simulink model "mobilebot_Model"  (R2018a)
settings: Solver=VariableStepAuto  StartTime=0.0  StopTime=10.0  RelTol=1e-3
libraries: simulink x2
settings Model: Creator=ewolbrec  LastModifiedBy=nalha
settings CodeAppCC: StateflowObjectComments=on

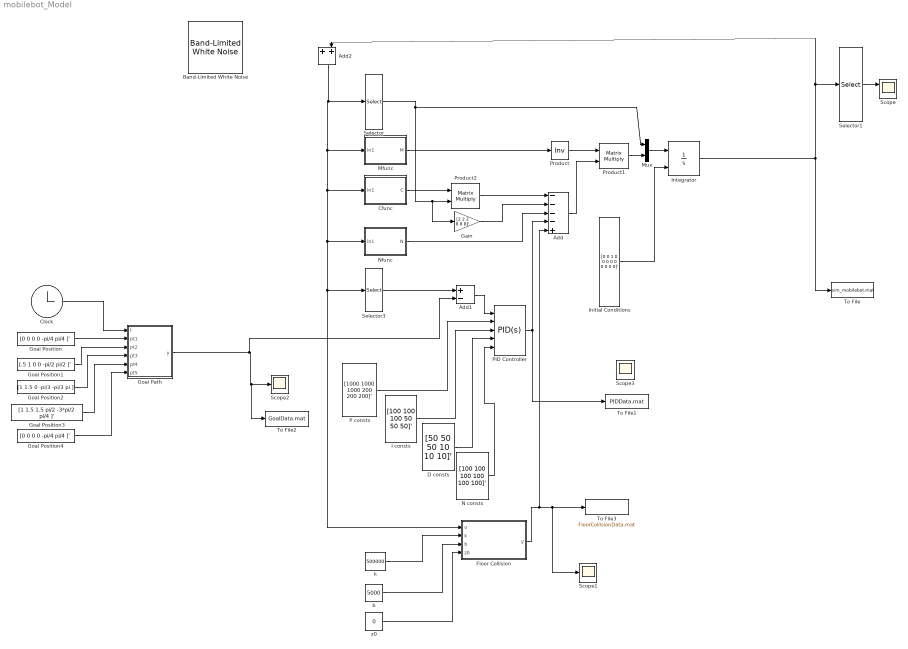
== system mobilebot_Model ==
  Add : Sum  Inputs=----+
  Add1 : Sum  Inputs=+-
  Add2 : Sum
  Band-Limited White Noise : simulink/Sources/Band-Limited White Noise  Cov=[0.00001 0.00001 0.0 0.00001 0.00001 0.00001 0.00001 0.00001 0.00001 0.00001 0.00001 0.00001]  Ts=1/30  seed=[23341 45275 30585 21083 69043 57234 42583 21474 10234 94373 48378 902740]
  Cfunc : MATLAB Function  TreatAsAtomicUnit=on
  Clock : Clock
  D consts : Constant  Value=[50 50 50 10 10 10]'  VectorParams1D=off
  Floor Collision : MATLAB Function  TreatAsAtomicUnit=on
  Gain : Gain  Gain=[2 2 2 8 8 8]'
  Goal Path : MATLAB Function  TreatAsAtomicUnit=on
  Goal Position : Constant  Value=[0 0 0 0 -pi/4 pi/4 ]'  VectorParams1D=off
  Goal Position1 : Constant  Value=[.5 1 0 0 -pi/2 pi/2 ]'  VectorParams1D=off
  Goal Position2 : Constant  Value=[1 1.5 0 -pi/3 -pi/3 pi ]'  VectorParams1D=off
  Goal Position3 : Constant  Value=[1 1.5 1.5 pi/2 -3*pi/2 pi/4 ]'  VectorParams1D=off
  Goal Position4 : Constant  Value=[0 0 0 0 -pi/4 pi/4 ]'  VectorParams1D=off
  I consts : Constant  Value=[100 100 100 50 50 50]'  VectorParams1D=off
  Initial Conditions : Constant  Value=[0 0 1 0 0 0 0 0 0 0 0 0]'  VectorParams1D=off
  Integrator : Integrator  InitialConditionSource=external
  Mfunc : MATLAB Function  TreatAsAtomicUnit=on
  Mux : Mux  Inputs=2
  N consts : Constant  Value=[100 100 100 100 100 100]'  VectorParams1D=off
  Nfunc : MATLAB Function  TreatAsAtomicUnit=on
  P consts : Constant  Value=[1000 1000 1000 200 200 200]'  VectorParams1D=off
  PID Controller : simulink/Continuous/PID Controller  Controller=PID  TimeDomain=Continuous-time  SampleTime=-1  IntegratorMethod=Forward Euler  FilterMethod=Forward Euler  Form=Parallel  UseFilter=on  ControllerParametersSource=external  P=200  I=25  D=70  N=150  InitialConditionSource=internal  InitialConditionForIntegrator=0  InitialConditionForFilter=0  ExternalReset=none  LimitOutput=off  UpperSaturationLimit=inf  LowerSaturationLimit=-inf  LinearizeAsGain=on  AntiWindupMode=none  Kb=1  TrackingMode=off  Kt=1  PParamMin=[]  PParamMax=[]  IParamMin=[]  IParamMax=[]  DParamMin=[]  DParamMax=[]  NParamMin=[]  NParamMax=[]  KbParamMin=[]  KbParamMax=[]  KtParamMin=[]  KtParamMax=[]  POutMin=[]  POutMax=[]  IOutMin=[]  IOutMax=[]  DOutMin=[]  DOutMax=[]  NOutMin=[]  NOutMax=[]  KbOutMin=[]  KbOutMax=[]  KtOutMin=[]  KtOutMax=[]  IntegratorOutMin=[]  IntegratorOutMax=[]  FilterOutMin=[]  FilterOutMax=[]  SumOutMin=[]  SumOutMax=[]  SumI1OutMin=[]  SumI1OutMax=[]  SumI2OutMin=[]  SumI2OutMax=[]  SumI3OutMin=[]  SumI3OutMax=[]  SumDOutMin=[]  SumDOutMax=[]  SaturationOutMin=[]  SaturationOutMax=[]  IntegratorContinuousStateAttributes=''  IntegratorStateMustResolveToSignalObject=off  IntegratorRTWStateStorageClass=Auto  FilterContinuousStateAttributes=''  FilterStateMustResolveToSignalObject=off  FilterRTWStateStorageClass=Auto  DifferentiatorICPrevScaledInput=0  DifferentiatorOutMin=[]  DifferentiatorOutMax=[]  FilterDiffOutCoefMin=[]  FilterDiffOutCoefMax=[]  SumDenOutMin=[]  SumDenOutMax=[]  SumNumOutMin=[]  SumNumOutMax=[]  ReciprocalOutMin=[]  ReciprocalOutMax=[]  DivideOutMin=[]  DivideOutMax=[]  TunerSelectOption=Transfer Function Based (PID Tuner App)
  Product : Product  Inputs=/  Multiplication=Matrix(*)
  Product1 : Product  Inputs=**  Multiplication=Matrix(*)
  Product2 : Product  Inputs=**  Multiplication=Matrix(*)
  Scope : Scope  NumInputPorts=2
  Scope1 : Scope
  Scope2 : Scope
  Scope3 : Scope
  Selector : Selector  InputPortWidth=12  IndexOptions=Index vector (dialog)  Indices=[7 8 9 10 11 12]  OutputSizes=1
  Selector1 : Selector  InputPortWidth=12  IndexOptions=Index vector (dialog)  Indices=[1 2 3 4 5 6]  OutputSizes=1
  Selector3 : Selector  InputPortWidth=12  IndexOptions=Index vector (dialog)  Indices=[1 2 3 4 5 6]  OutputSizes=1
  To File : ToFile  Filename=sim_mobilebot.mat  SampleTime=1/30
  To File1 : ToFile  Filename=PIDData.mat  SampleTime=1/30
  To File2 : ToFile  Filename=GoalData.mat  SampleTime=1/30
  To File3 : ToFile  Filename=FloorCollisionData.mat  SampleTime=1/30
  "b " : Constant  Value=5000
  "k " : Constant  Value=500000
  z0 : Constant  Value=0
  wires:
  Mfunc/1(M) -> Product/1
  Mux/1 -> Integrator/1
  Product1/1 -> Mux/2
  Selector/1 -> Gain/1, Product2/2, Mux/1
  Cfunc/1(C) -> Product2/1
  Product/1 -> Product1/1
  Gain/1 -> Add/2
  Product2/1 -> Add/1
  Nfunc/1(N) -> Add/3
  Add/1 -> Product1/2
  Initial Conditions/1 -> Integrator/2
  Selector1/1 -> Scope/1
  Selector3/1 -> Add1/1
  Add1/1 -> PID Controller/1
  Integrator/1 -> To File/1, Add2/2, Selector1/1
  PID Controller/1 -> To File1/1, Add/4
  Floor Collision/1(y) -> Scope1/1, To File3/1, Add/5
  "k "/1 -> Floor Collision/2(k)
  "b "/1 -> Floor Collision/3(b)
  z0/1 -> Floor Collision/4(z0)
  P consts/1 -> PID Controller/2
  I consts/1 -> PID Controller/3
  D consts/1 -> PID Controller/4
  Clock/1 -> Goal Path/1(t)
  Goal Position/1 -> Goal Path/2(pt1)
  Goal Position1/1 -> Goal Path/3(pt2)
  Goal Position2/1 -> Goal Path/4(pt3)
  Goal Position3/1 -> Goal Path/5(pt4)
  Goal Position4/1 -> Goal Path/6(pt5)
  Goal Path/1(y) -> Add1/2, To File2/1, Scope2/1
  N consts/1 -> PID Controller/5
  Add2/1 -> Mfunc/1(in1), Cfunc/1(in1), Nfunc/1(in1), Selector3/1, Floor Collision/1(u), Selector/1

== matlab function mobilebot_Model/Cfunc ==
  data: in1 input; C output
function C = Cfunc(in1)
%#codegen

%    This function was generated by the Symbolic Math Toolbox version 8.1.
%    10-May-2018 12:26:45

th4 = in1(4,:);
th5 = in1(5,:);
th6 = in1(6,:);
th4d = in1(10,:);
th5d = in1(11,:);
th6d = in1(12,:);
t2 = cos(th4);
t3 = cos(th5);
t4 = sin(th4);
t5 = cos(th6);
t6 = sin(th5);
t7 = sin(th6);
t8 = t2.*t3.*t7.*th4d.*(2.7e1./8.0);
t9 = t2.*t5.*t6.*th4d.*(2.7e1./8.0);
t10 = t3.*t4.*t5.*th5d.*(2.7e1./8.0);
t11 = t3.*t4.*t5.*th6d.*(2.7e1./8.0);
t12 = t3.*t4.*t7.*th4d.*(2.7e1./8.0);
t13 = t4.*t5.*t6.*th4d.*(2.7e1./8.0);
t14 = t2.*t6.*t7.*th5d.*(2.7e1./8.0);
t15 = t2.*t6.*t7.*th6d.*(2.7e1./8.0);
t16 = th5+th6;
t17 = sin(t16);
t18 = th5.*2.0;
t19 = th6.*2.0;
t20 = t18+t19;
t21 = sin(t20);
t22 = t18+th6;
t23 = sin(t22);
t24 = sin(t18);
t25 = cos(t16);
t26 = th5d+th6d;
t27 = t21.*3.3e1;
C = reshape([0.0,0.0,0.0,0.0,0.0,0.0,0.0,0.0,0.0,0.0,0.0,0.0,0.0,0.0,0.0,0.0,0.0,0.0,t2.*th4d.*(5.13e2./1.0e2)+t3.*t4.*th4d.*(8.1e1./8.0)+t2.*t6.*th5d.*(8.1e1./8.0)+t3.*t4.*t5.*th4d.*(2.7e1./8.0)+t2.*t3.*t7.*th5d.*(2.7e1./8.0)+t2.*t3.*t7.*th6d.*(2.7e1./8.0)+t2.*t5.*t6.*th5d.*(2.7e1./8.0)+t2.*t5.*t6.*th6d.*(2.7e1./8.0)-t4.*t6.*t7.*th4d.*(2.7e1./8.0),t4.*th4d.*(5.13e2./1.0e2)-t2.*t3.*th4d.*(8.1e1./8.0)+t4.*t6.*th5d.*(8.1e1./8.0)-t2.*t3.*t5.*th4d.*(2.7e1./8.0)+t2.*t6.*t7.*th4d.*(2.7e1./8.0)+t3.*t4.*t7.*th5d.*(2.7e1./8.0)+t3.*t4.*t7.*th6d.*(2.7e1./8.0)+t4.*t5.*t6.*th5d.*(2.7e1./8.0)+t4.*t5.*t6.*th6d.*(2.7e1./8.0),0.0,t7.*th6d.*(-2.7e1./3.2e1)-t21.*th5d.*5.56875e-1-t21.*th6d.*5.56875e-1-t23.*th5d.*(2.7e1./1.6e1)-t23.*th6d.*(2.7e1./3.2e1)-t24.*th5d.*2.244375,th4d.*(t23.*1.0e2+t24.*1.33e2+t27).*1.6875e-2,th4d.*(t7.*5.0e1+t23.*5.0e1+t27).*1.6875e-2,t8+t9+t10+t11+t2.*t6.*th4d.*(8.1e1./8.0)+t3.*t4.*th5d.*(8.1e1./8.0)-t4.*t6.*t7.*th5d.*(2.7e1./8.0)-t4.*t6.*t7.*th6d.*(2.7e1./8.0),t12+t13+t14+t15-t2.*t3.*th5d.*(8.1e1./8.0)+t4.*t6.*th4d.*(8.1e1./8.0)-t2.*t3.*t5.*th5d.*(2.7e1./8.0)-t2.*t3.*t5.*th6d.*(2.7e1./8.0),t6.*th5d.*(8.1e1./8.0)+t17.*th5d.*(2.7e1./8.0)+t17.*th6d.*(2.7e1./8.0),t3.*th5d.*(-8.1e1./1.6e2)-t21.*th4d.*5.56875e-1-t23.*th4d.*(2.7e1./1.6e1)-t24.*th4d.*2.244375-t25.*th5d.*(2.7e1./1.6e2)-t25.*th6d.*(2.7e1./1.6e2),t7.*th6d.*(-2.7e1./1.6e1),t7.*th5d.*(2.7e1./1.6e1),t8+t9+t10+t11-t4.*t6.*t7.*th5d.*(2.7e1./8.0)-t4.*t6.*t7.*th6d.*(2.7e1./8.0),t12+t13+t14+t15-t2.*t3.*t5.*th5d.*(2.7e1./8.0)-t2.*t3.*t5.*th6d.*(2.7e1./8.0),t17.*t26.*(2.7e1./8.0),t7.*th4d.*(-2.7e1./3.2e1)-t21.*th4d.*5.56875e-1-t23.*th4d.*(2.7e1./3.2e1)-t25.*th5d.*(2.7e1./1.6e2)-t25.*th6d.*(2.7e1./1.6e2),t7.*t26.*(-2.7e1./1.6e1),0.0],[6,6]);

== matlab function mobilebot_Model/Mfunc ==
  data: in1 input; M output
function M = Mfunc(in1)
%#codegen

%    This function was generated by the Symbolic Math Toolbox version 8.1.
%    10-May-2018 12:26:45

th4 = in1(4,:);
th5 = in1(5,:);
th6 = in1(6,:);
t2 = cos(th4);
t3 = cos(th5);
t4 = sin(th4);
t5 = sin(th5);
t6 = th5+th6;
t7 = sin(t6);
t8 = sin(th6);
t9 = cos(th6);
t10 = t5.*3.0;
t11 = t7+t10;
t12 = cos(t6);
t13 = t4.*(5.13e2./1.0e2);
t14 = t2.*t5.*t8.*(2.7e1./8.0);
t15 = t13+t14-t2.*t3.*(8.1e1./8.0)-t2.*t3.*t9.*(2.7e1./8.0);
t16 = t4.*t5.*t8.*(2.7e1./8.0);
t17 = t2.*(-5.13e2./1.0e2)+t16-t3.*t4.*(8.1e1./8.0)-t3.*t4.*t9.*(2.7e1./8.0);
t18 = th5.*2.0;
t19 = t4.*t11.*(2.7e1./8.0);
t24 = t12.*(2.7e1./8.0);
t20 = t3.*(-8.1e1./8.0)-t24;
t25 = t7.*(2.7e1./1.6e2);
t21 = t5.*(-8.1e1./1.6e2)-t25;
t22 = t9.*(2.7e1./1.6e1);
t23 = t4.*t7.*(2.7e1./8.0);
t26 = t22+9.07e2./8.0e2;
M = reshape([7.83e2./5.0,0.0,0.0,t15,t19,t23,0.0,7.83e2./5.0,0.0,t17,t2.*t11.*(-2.7e1./8.0),t2.*t7.*(-2.7e1./8.0),0.0,0.0,7.83e2./5.0,0.0,t20,-t24,t15,t17,0.0,t22+cos(t18+th6.*2.0).*5.56875e-1+cos(t18+th6).*(2.7e1./1.6e1)+cos(t18).*2.244375+6.69275,t21,-t25,t19,t2.*t11.*(-2.7e1./8.0),t20,t21,t9.*(2.7e1./8.0)+5.6425,t26,t23,t2.*t7.*(-2.7e1./8.0),t12.*(-2.7e1./8.0),t7.*(-2.7e1./1.6e2),t26,9.07e2./8.0e2],[6,6]);

== matlab function mobilebot_Model/Nfunc ==
  data: in1 input; N output
function N = Nfunc(in1)
%#codegen

%    This function was generated by the Symbolic Math Toolbox version 8.1.
%    10-May-2018 12:26:45

th5 = in1(5,:);
th6 = in1(6,:);
t2 = th5+th6;
t3 = cos(t2);
N = [0.0;0.0;1.566e3;0.0;t3.*(-1.35e2./4.0)-cos(th5).*(4.05e2./4.0);t3.*(-1.35e2./4.0)];

== matlab function mobilebot_Model/Floor Collision ==
  data: u input; y output; k input; b input; z0 input
function y = floorSpringDamper(u, k, b, z0)

y = zeros(6,1); %set output equal to zero

if u(3) < z0 % if we're below z0
    
    y(3) = -k*(u(3)-z0) - b*u(9); %spring + damper force response
    
end

== matlab function mobilebot_Model/Goal Path ==
  data: t input; y output; pt1 input; pt2 input; pt3 input; pt4 input; pt5 input
function y = path(t, pt1, pt2, pt3, pt4, pt5)
% Generate current desired position as defined in this path function
y = zeros(6,1);
tlength = linspace(0, 10, 5);
pt = [pt1 pt2 pt3 pt4 pt5];
p1 = polyfit(tlength,pt(1,:),4);
p2 = polyfit(tlength,pt(2,:),4);
p3 = polyfit(tlength,pt(3,:),4);
p4 = polyfit(tlength,pt(4,:),4);
p5 = polyfit(tlength,pt(5,:),4);
p6 = polyfit(tlength,pt(6,:),4);


y = [   polyval(p1,t);
        polyval(p2,t);
        polyval(p3,t);
        polyval(p4,t);
        polyval(p5,t);
        polyval(p6,t)];

% 
% if t < 2
%     y = pt1 .* (0.2*t);
%     %[pt1(1)*.2*t pt1(2)*.2*t pt1(3)*.2*t pt1(4)*.2*t pt1(5)*.2*t pt1(6)*.2*t]';
% end
% 
% if t > 2 && t < 4
%     y = pt2 .* (0.2*(t-2));
% end
% 
% if t > 4 && t < 6
%     y = pt3 .* (0.2*(t-4));
% end
% 
% if t > 6 && t < 8
%     y = pt4 .* (0.2*(t-6));
% end
% 
% if t > 8 && t < 10
%     y = pt5 .* (0.2*(t-8));
% end
%y = [.2*t -.2*t .2*t -(pi/32)*t (pi/32)*t (pi/32)*t]';
